simulink model "rtlsdr_am_ssb_demod"  (R2014b)
settings: Solver=ode45  StartTime=0.0  StopTime=60  RelTol=1e-3
PreLoadFcn:
  | %%%%%%%%%%%%%%%%%%%%%%%%%%%%%%%%%%%%%%%%%%%%%%%%%%%%%%%%%%%%%%%%%%%%%%%%%%%
  | % check to see if Simulink library folder is missing from the MATLAB path %
  | %%%%%%%%%%%%%%%%%%%%%%%%%%%%%%%%%%%%%%%%%%%%%%%%%%%%%%%%%%%%%%%%%%%%%%%%%%%
  | if isempty(strfind(path, 'rtlsdr_book_library'))
  | 
  |     % create error window
  |     fig_error = figure(...
  |         'Name', 'Error: RTL-SDR Book Library',...
  |         'Toolbar','none',...
  |         'MenuBar','none',...
  |         'NumberTitle','off',...
  |         'Resize','off',...
  |         'WindowStyle','modal');
  |     fig_error.Position(3) = 600;
  |     fig_error.Position(4) = 150;
  |     fig_axes = axes(...
  |         'Parent',fig_error,...
  |         'Position',[0,0,1,1],...
  |         'visible','off');
  |     % error message
  |     t_title = text(.05,.8,...
  |         'MISSING DIRECTORIES',...
  |         'FontSize',11.5);
  |     t_body = text(.075,.6,...
  |         [{'Simulink cannot find the  \it{<root>}\rm / \it{rtlsdr\_book\_library}\rm  folder in the \it{MATLAB Path}\rm.'},...
  |         {'Please set the MATLAB path following the instructions given in Exercise 2.4.'}],...
  |         'FontSize',10.5);
  |     % buttons
  |     btn_path = uicontrol(...
  |         'Parent',fig_error,...
  |         'String','Set Path Now',...
  |         'FontSize',10,...
  |         'Callback', 'pathtool; close(fig_error);',...
  |         'Position', [fig_error.Position(3)/2-210, 30, 200, 30]);
  |     btn_abort = uicontrol(...
  |         'Parent',fig_error,...
  |         'String','No thanks',...
  |         'FontSize',10,...
  |         'Callback', 'close(fig_error); abort=1;',...
  |         'Position', [fig_error.Position(3)/2+10, 30, 200, 30]);
  | 
  |     % pause to allow user to interact with error box
  |     uiwait(fig_error);
  | 
  |     % abort simulation
  |     try
  |         if abort==1
  |             set_param(gcs, 'SimulationCommand', 'stop');
  |         end
  |     end
  | 
  |     % if user has set path, allow diagram to be updated
  |     if ~exist('abort','var')
  |         % create error window
  |         fig_update = figure(...
  |             'Name', 'Update Diagram',...
  |             'Toolbar','none',...
  |             'MenuBar','none',...
  |             'NumberTitle','off',...
  |             'Resize','off');
  |         fig_update.Position(3) = 400;
  |         fig_update.Position(4) = 120;
  |         fig_axes = axes(...
  |             'Parent',fig_update,...
  |             'Position',[0,0,1,1],...
  |             'visible','off');
  |         % instruction message
  |         t_body = text(.075,.7,...
  |             'Once you have set the path, update the block diagram',...
  |             'FontSize',10.5);
  |         % button
  |         btn_update = uicontrol(...
  |             'Parent',fig_update,...
  |             'String','Update Block Diagram',...
  |             'FontSize',10,...
  |             'Callback', 'set_param(gcs,''SimulationCommand'',''update''); close(gcf)',...
  |             'Position', [fig_update.Position(3)/2-100, 30, 200, 30]);
  |     end
  | 
  |     % clear error components
  |     clear('fig_error','fig_update','fig_axes','t_title','t_body','btn_path','btn_abort','btn_update','abort');
  | 
  | end
  | %%%%%%%%%%%%%%%%%%%%%%%%%%%%%%%%%%%%%%%%%%%%%%%%%%%%%%%%%%%%%%%%%%%%%%%%%%%
undefined symbols (not defined in the file or in its folder): dfilt, fdesignblkfcn, gcbh, startfcn_spectrum_analyzer
libraries: dspsrcs4 x2, rtlsdr_book_library x2, dspmlti4 x1, dsparch4 x1, sdrrlib x1, dspsnks4 x1
CloseFcn:
  | closefcn_model;
Description:
  | Software, Simulation Examples and Design Exercises Licence Agreement
  | 
  | This license agreement refers to the simulation examples, design exercises and files,
  | and associated software MATLAB and Simulink resources that accompany the book:
  | 
  |      Title: Software Defined Radio using MATLAB & Simulink and the RTL-SDR
  |      Published by Strathclyde Academic Media, 2015
  |      Authored by Robert W. Stewart, Kenneth W. Barlee, Dale S.W. Atkinson,
  |      and Louise H. Crockett
  | 
  | and made available as a download from, www.desktopSDR.com or variously acquired
  | by other means such as via USB storage, cloud storage, disk or any other electronic
  | or optical or magnetic storage mechanism. These files and associated software may
  | be used subject to the terms of agreement of the conditions below:
  | 
  |     Copyright © 2015 Robert W. Stewart, Kenneth W. Barlee, Dale S.W. Atkinson,
  |     and Louise H. Crockett
  |     All rights reserved.
  | 
  | Redistribution and use in source and binary forms, with or without modification, are
  | permitted provided that the following conditions are met:
  | 
  |    1.  Redistributions of source code must retain the above copyright notice, this list of
  |         conditions and the following disclaimer.
  | 
  |    2.  Redistributions in binary form must reproduce the above copyright notice, this
  |         list of conditions and the following disclaimer in the documentation and/or other
  |         materials provided with the distribution.
  | 
  |    3.  Neither the name of the copyright holder nor the names of its contributors may
  |         be used to endorse or promote products derived from this software without
  |         specific prior written permission.
  | 
  |    4.  In all cases, the software is, and all modifications and derivatives of the
  |         software shall be, licensed to you solely for use in conjunction with The
  |         MathWorks, Inc. products and service offerings.
  | 
  | THIS SOFTWARE IS PROVIDED BY THE COPYRIGHT HOLDERS AND CONTRIBUTORS
  | "AS IS" AND ANY EXPRESS OR IMPLIED WARRANTIES, INCLUDING, BUT NOT LIMITED
  | TO, THE IMPLIED WARRANTIES OF MERCHANTABILITY AND FITNESS FOR A
  | PARTICULAR PURPOSE ARE DISCLAIMED. IN NO EVENT SHALL THE COPYRIGHT
  | HOLDER OR CONTRIBUTORS BE LIABLE FOR ANY DIRECT, INDIRECT, INCIDENTAL,
  | SPECIAL, EXEMPLARY, OR CONSEQUENTIAL DAMAGES (INCLUDING, BUT NOT
  | LIMITED TO, PROCUREMENT OF SUBSTITUTE GOODS OR SERVICES; LOSS OF USE,
  | DATA, OR PROFITS; OR BUSINESS INTERRUPTION) HOWEVER CAUSED AND ON ANY
  | THEORY OF LIABILITY, WHETHER IN CONTRACT, STRICT LIABILITY, OR TORT
  | (INCLUDING NEGLIGENCE OR OTHERWISE) ARISING IN ANY WAY OUT OF THE USE
  | OF THIS SOFTWARE, EVEN IF ADVISED OF THE POSSIBILITY OF SUCH DAMAGE.
  | 
  | 
  | Audio Tracks used in Simulations Examples and Design Exercises
  | 
  | The music and vocal files used within the Examples files and software within the book
  | were variously written, arranged, performed, recorded and produced by Garrey Rice,
  | Adam Struth, Jamie Struth, Iain Thistlethwaite and also Marshall Craigmyle who
  | collectively, and individually where appropriate, assert and retain all of their copyright,
  | performance and artistic rights. Permission to use and reproduce this music is
  | granted for all purposes associated with MATLAB and Simulink software and the
  | simulation examples and design exercises files that accompany this book. Requests to
  | use the music for any other purpose should be directed to: info@desktopSDR.com.
  | For information on music track names, full credits, and links to the musicians please
  | refer to www.desktopSDR.com/more/audio.
settings Model: SimulationMode=accelerator  Creator=desktopSDR Team  LastModifiedBy=desktopSDR Team
settings DataIOCC: LimitDataPoints=off  SaveOutput=off  SignalLogging=off  SaveTime=off
settings OptimizationCC: EfficientMapNaN2IntZero=off
settings HardwareCC: TargetLongLongMode=on  TargetIntDivRoundTo=Zero  TargetEndianess=LittleEndian  TargetHWDeviceType=MATLAB Host  ProdEqTarget=off
settings CodeAppCC: MaxIdLength=128
settings GRTTargetCC: CombineOutputUpdateFcns=off  GRTInterface=on

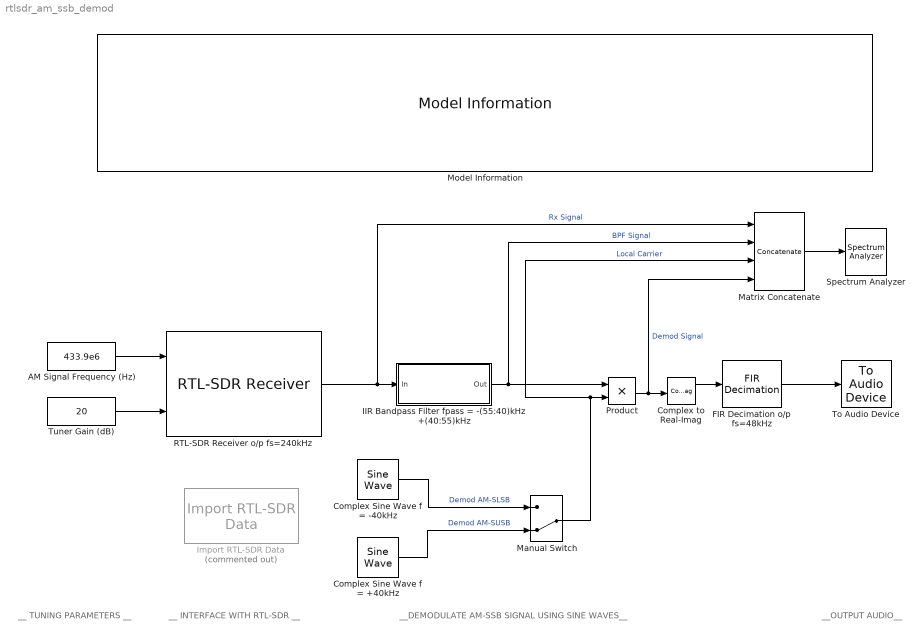
== system rtlsdr_am_ssb_demod ==
  note: __ TUNING PARAMETERS __
  note: __ INTERFACE WITH RTL-SDR __
  note: __OUTPUT AUDIO__
  note: __DEMODULATE AM-SSB SIGNAL USING SINE WAVES__
  AM Signal Frequency (Hz) : Constant  Value=433.9e6
  Complex Sine Wave f = +40kHz : dspsrcs4/Sine Wave  Amplitude=1  Frequency=40e3  Phase=0  SampleMode=Discrete  OutComplex=Complex  CompMethod=Trigonometric fcn  TableSize=Speed  SampleTime=1/240e3  SamplesPerFrame=4096  ResetState=Restart at time zero  dataType=single  wordLen=16  udDataType=sfix(16)  fracBitsMode=Best precision  numFracBits=15  OutDataTypeStr=single  LastOutDataTypeStr=single
  Complex Sine Wave f = -40kHz : dspsrcs4/Sine Wave  Amplitude=1  Frequency=-40e3  Phase=0  SampleMode=Discrete  OutComplex=Complex  CompMethod=Trigonometric fcn  TableSize=Speed  SampleTime=1/240e3  SamplesPerFrame=4096  ResetState=Restart at time zero  dataType=single  wordLen=16  udDataType=sfix(16)  fracBitsMode=Best precision  numFracBits=15  OutDataTypeStr=single  LastOutDataTypeStr=single
  Complex to Real-Imag : ComplexToRealImag
  FIR Decimation o/p fs=48kHz : dspmlti4/FIR Decimation  h=firpm(100, [0 15e3 20e3 (240e3/2)]/(240e3/2), [1 1 0 0], [1 1], 20)  D=5  filtStruct=Direct form  framing=Allow multirate processing  inputOffset=0  outputBufInitCond=0  InputProcessing=Columns as channels (frame based)  firstCoeffDataTypeStr=Inherit: Same word length as input  firstCoeffLastDataTypeStr=Inherit: Same word length as input  firstCoeffMin=[]  firstCoeffMax=[]  outputDataTypeStr=Inherit: Same as accumulator  outputLastDataTypeStr=Inherit: Same as accumulator  outputMin=[]  outputMax=[]  roundingMode=Floor  overflowMode=off  FilterSource=Specify via dialog  FilterObject=Hm_firdecim
      settings: allowOverrides=off
  IIR Bandpass Filter fpass = -(55:40)kHz +(40:55)kHz : Subsystem  DialogController=fdesignblkfcn  InitFcn=fdesignblkfcn(gcbh, {'InitFcn'});  mask(Bandpass Filter){}
      mask help: Design a bandpass filter
      settings: CopyFcn=fdesignblkfcn(gcbh, {'CopyFcn'});
      mask Help: helpview(mapfilelocation('dsp'), 'dspbandpassfilter');
      mask Display: disp('Bandpass');
  Import RTL-SDR Data : rtlsdr_book_library/Additional Tools/Import RTL-SDR Data  Commented=on  filename=rec_data/am_ssb.mat  frm_size=4096  data_type=single
  Manual Switch : ManualSwitch  CurrentSetting=0
  Matrix Concatenate : Concatenate  NumInputs=4  Mode=Multidimensional array  ConcatenateDimension=2
  Model Information : rtlsdr_book_library/Additional Tools/Model Information/Model Information
  Product : Product
  RTL-SDR Receiver o/p fs=240kHz : sdrrlib/RTL-SDR Receiver  SourceLibraryInfo="This block requires <a href=\"http://www.mathworks.com/hardware-support/rtl-sdr.html\">Communications System Toolbox Support Package for RTL-SDR Radio</a>"  sobjType=sdrr.internal.SDRRTLReceiverSL  IPAddress=0  dataUDPPort=-1  ctrlUDPPort=-1  subDeviceList=nosubdev  sdrBlockType=SDRBlockTypeSLT.SDRRxBlock  requester=UNUSED_BY_SFCN  sdrExecutionMode=SDRExecutionModeSLT.ExecModeHW  LostSamplesOutputPort=off  OutputDataType=single  FrameLength=4096  EnableBurstMode=off  NumFramesInBurst=20  BypassUserLogic=off  DecimatorSelect=DDC decimator  SourceSelect=RF data  SineAmplitude=16000  EnableInternalClock=off  BypassIQBalance=off  CenterFrequency=433.9e6-100e3  IFBandwidth=40e6  ADCRateSource=Dialog  ADCRate=240e3  CenterFrequencySource=Input port  GainSource=Input port  IntermediateFrequency=0  Gain=40  DecimationFactorSource=Dialog  DecimationFactor=512  RFFrequencyIsTunable=logical(1)  SampleTime=(4096)/(240e3)  IFBandwidthSource=Dialog  SineFrequency=30000  BypassDCBlockingFilter=off  IntermediateFrequencySource=Dialog  IQBalanceCoefficients=64  SkipAllHardwareResetAndInitialization=off  EnableIQCalibrationTable=on  CacheIQCalibrationTable=off  EnableOffsetTuning=off  EnableRTLAGC=off  EnableTestMode=off  EnableTunerAGC=off  FrequencyCorrectionSource=Dialog  FrequencyCorrection=0  NumMLBuffers=128  NumUSBBuffers=16  LatencyOutputPort=off  RTLCrystalFrequency=28800000  TunerCrystalFrequency=28800000
  Spectrum Analyzer : SpectrumAnalyzer  StartFcn=startfcn_spectrum_analyzer;
  To Audio Device : dspsnks4/To Audio Device  deviceName=Default  inheritSampleRate=on  sampleRate=44100  deviceDatatype=Determine from input data type  autoBufferSize=on  bufferSize=4096  queueDuration=1.0  defaultOutputChannelMapping=on  outputChannelMapping=1  outputNumUnderrunSamples=off
  Tuner Gain (dB) : Constant  Value=20
  wires:
  Matrix Concatenate/1 -> Spectrum Analyzer/1
  Manual Switch/1 -> Matrix Concatenate/3, Product/2  "Local Carrier"
  AM Signal Frequency (Hz)/1 -> RTL-SDR Receiver o/p fs=240kHz/1
  Tuner Gain (dB)/1 -> RTL-SDR Receiver o/p fs=240kHz/2
  Product/1 -> Matrix Concatenate/4, Complex to Real-Imag/1  "Demod Signal"
  FIR Decimation o/p fs=48kHz/1 -> To Audio Device/1
  IIR Bandpass Filter fpass = -(55:40)kHz +(40:55)kHz/1(Out) -> Product/1, Matrix Concatenate/2  "BPF Signal"
  Complex to Real-Imag/1 -> FIR Decimation o/p fs=48kHz/1
  Complex Sine Wave f = +40kHz/1 -> Manual Switch/2  "Demod AM-SUSB"
  Complex Sine Wave f = -40kHz/1 -> Manual Switch/1  "Demod AM-SLSB"
  RTL-SDR Receiver o/p fs=240kHz/1 -> IIR Bandpass Filter fpass = -(55:40)kHz +(40:55)kHz/1(In), Matrix Concatenate/1  "Rx Signal"

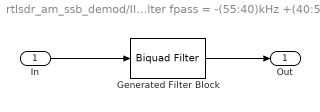
== system rtlsdr_am_ssb_demod/IIR Bandpass Filter fpass = -(55:40)kHz +(40:55)kHz ==
  In : Inport
  Generated Filter Block : dsparch4/Biquad Filter  Tag=BlockMethodSubSystem  IIRFiltStruct=Direct form II  CoeffSource=Specify via dialog  BiQuadCoeffs=[0.42214887875549534 0 -0.42214887875549534 1 -0.98823865611538131 0.97401451420547847;0.033061818692291765 0 -0.033061818692291765 1 -0.255562987775724 0.97029176883907564;0.40962932940897723 0 -0.40962932940897723 1 -0.96374853338649646 0.93400621778983428;0.061627256862270989 0 -0.061627256862270989 1 -0.25549067244038548 0.92491042766383424;0.34804686769186149 0 -0.34804686769186149 1 -0.25882003299069856 0.89279954523166905;0.074485120089956947 0 -0.074485120089956947 1 -0.9294141511065368 0.88695355833419864;0.3380356932077454 0 -0.3380356932077454 1 -0.26749175946597026 0.85279211642514474;0.11414706942811309 0 -0.11414706942811309 1 -0.8993097642364567 0.85187677749258039;0.26975453210172951 0 -0.26975453210172951 1 -0.86713478372906905 0.8192510152074981;0.15169389058649052 0 -0.15169389058649052 1 -0.28068513798157396 0.8162190780957822;0.23486896109857225 0 -0.23486896109857225 1 -0.8331265846567526 0.78923822131355625;0.12543246219034992 0 -0.12543246219034992 1 -0.29806112006699154 0.78328747888967065;0.30344638398123625 0 -0.30344638398123625 1 -0.31363630953671184 0.7610844489222911;0.14204372882356484 0 -0.14204372882356484 1 -0.7883970800288258 0.75566031393796895;0.29204059077048644 0 -0.29204059077048644 1 -0.337525516067535 0.7349293069292292;0.15769964715736565 0 -0.15769964715736565 1 -0.75113712047955783 0.73217586967172454;0.28024335208989254 0 -0.28024335208989254 1 -0.36467175756862613 0.71283395976825903;0.26861034304041859 0 -0.26861034304041859 1 -0.71285267464898394 0.71190933155127689;0.17198129605653537 0 -0.17198129605653537 1 -0.67383770529027076 0.69506646138757555;0.25591667733589984 0 -0.25591667733589984 1 -0.39472573928461274 0.69490448416156714;0.18545503193518079 0 -0.18545503193518079 1 -0.63441698320262108 0.68185149992041572;0.24243607863414046 0 -0.24243607863414046 1 -0.42732343258114791 0.68121939209674687;0.19746276667054932 0 -0.19746276667054932 1 -0.5949462076194667 0.67245728159958573;0.22744846625978013 0 -0.22744846625978013 1 -0.46208364928113799 0.67182458166320957;0.20641989162778182 0 -0.20641989162778182 1 -0.55580817687549611 0.6670545864829549;0.21354369604454937 0 -0.21354369604454937 1 -0.49860880019001874 0.66672790281337901;0.19683387716962003 0 -0.19683387716962003 1 -0.5364892331149077 0.66589493968373292;0.18908777013081096 0 -0.18908777013081096 1 -0.51740549209822551 0.66578232446690089;0.1666062095253458 0 -0.1666062095253458 1 -0.57531079591545409 0.66924746270652935;0.17778848871060463 0 -0.17778848871060463 1 -0.48015100336670025 0.66874010197490674;0.16332726070194734 0 -0.16332726070194734 1 -0.61466449153557434 0.67666548406438465;0.17641184163212795 0 -0.17641184163212795 1 -0.44445772378311499 0.67598426002862111;0.16322683649562625 0 -0.16322683649562625 1 -0.6541565310644416 0.68799304779764836;0.15881803755463447 0 -0.15881803755463447 1 -0.41073003572575306 0.68752769149224158;0.18237880602184384 0 -0.18237880602184384 1 -0.37935764524482984 0.70334288149802093;0.15785452243334397 0 -0.15785452243334397 1 -0.69341695014314575 0.70304702878325664;0.18573995463450585 0 -0.18573995463450585 1 -0.35071303962816736 0.7233669329551885;0.15651735978372061 0 -0.15651735978372061 1 -0.73210527943577131 0.72162757090000862;0.19035218077552934 0 -0.19035218077552934 1 -0.32515241052156241 0.74750700407082749;0.18458592070356522 0 -0.18458592070356522 1 -0.76991241292530632 0.74352854068174234;0.17293280717418719 0 -0.17293280717418719 1 -0.81550826902422946 0.77526501687851923;0.16280924233707353 0 -0.16280924233707353 1 -0.80655855355071004 0.76854651729691692;0.19480307658196594 0 -0.19480307658196594 1 -0.85034522105691646 0.80390751919005965;0.16342802130064965 0 -0.16342802130064965 1 -0.2888713006732021 0.79928652585052429;0.20033951894213034 0 -0.20033951894213034 1 -0.88346607754879403 0.83524758637483043;0.17758411807395799 0 -0.17758411807395799 1 -0.27354455950918161 0.83406249088390871;0.19091925197822526 0 -0.19091925197822526 1 ...(+5189 chars)Flag=Warning  IC=0  ICnum=0  ICden=0  InputProcessing=Columns as channels (frame based)  denAccumFracLength=30  denProdOutputFracLength=30  secondMemoryFracLength=15  roundingMode=Floor  overflowMode=off  ScaleValues=[0.022496210801432579;1;1;1;1;1;1;1;1;1;1;1;1;1;1;1;1;1;1;1;1;1;1;1;1;1;1;1;1;1;1;1;1;1;1;1;1;1;1;1;1;1;1;1;1;1;1;1;1;1;1;1;1;1;1;1;1;1;1;1;1;1;1;1;1;1;1;1;1;1;1;1;1;1;1;1;1;1;1;1;1;1;1;1;1;1;1;1;1;1;1;1;1;1;1;1;1;1;1;1;1;1;1;1;1;1;1;1]  optimizeScaleValues=off  ScaleValueMode=Specify via input port (g)  scaleValueFracLength=14  FilterSource=Specify via dialog  dfiltObjectName=dfilt.df2tsos([1 0.3 0.4],[1 0.1 0.2])
  Out : Outport
  wires:
  Generated Filter Block/1 -> Out/1
  In/1 -> Generated Filter Block/1
